simulink model "controller"  (Simulink 7.5)
settings: Solver=FixedStepDiscrete  SolverMode=SingleTasking  StartTime=0.0  StopTime=10.0  FixedStep=0.01  RelTol=1e-3
InitFcn:
  | controller_params
undefined symbols (not defined in the file): C_d_sea_surge, d_prop, DiscIntNeverNeededParam, InitialPoint, IPStar, ISA_g, K_t, mass, MaxDwnPthStar, OC2max, phi_0, rho_w, switchDistance, tanIntercept, TStar, Turn2Track, wheelbase
libraries: simulink x8, uSimLib x3, aerolibconvert2 x2, simulink_need_slupdate x1
settings Model: Creator=Bryant  LastModifiedBy=Bryant
settings DataIOCC: LimitDataPoints=off  SaveOutput=off  SignalLogging=off  DSMLogging=off  SaveTime=off
settings OptimizationCC: InlineParams=on  InlineInvariantSignals=on  InitFltsAndDblsToZero=on  EfficientFloat2IntCast=on  SimCompilerOptimization=On
settings HardwareCC: ProdBitPerInt=16  ProdIntDivRoundTo=Zero  ProdEndianess=LittleEndian  ProdWordSize=16  ProdHWDeviceType=16-bit Generic
settings ModelReferenceCC: EnableParallelModelReferenceBuilds=on  ParallelModelReferenceMATLABWorkerInit=Copy Base Workspace  ModelReferenceNumInstancesAllowed=Single
settings RTWCC: SystemTargetFile=dspic.tlc  MakeCommand=make_CreateMPLAB  TemplateMakefile=dspic_pic30_gcc.tmf  PostCodeGenCommand=dsPIC_Compile()  Description=Embedded Target for Microchip dsPIC (real-time)  ProcessScript=dspic_make_rtw_hook
settings CodeAppCC: MaxIdLength=80
settings STFCustomTargetCC: IncludeMdlTerminateFcn=off  GeneratePreprocessorConditionals=Disable all  SupportNonInlinedSFcns=off  SystemTargetFile=dspic.tlc
settings ERTTargetCC: MultiwordLength=2048  ParMdlRefBuildCompliant=off  CompOptLevelCompliant=off  IncludeMdlTerminateFcn=off  GeneratePreprocessorConditionals=Disable all  CombineOutputUpdateFcns=off  ERTFirstTimeCompliant=off  ERTCustomFileBanners=off  SupportContinuousTime=on  ModelStepFunctionPrototypeControlCompliant=off  CPPClassGenCompliant=off  ExtModeMexFile=ext_serial_win32_comm  InlinedParameterPlacement=NonHierarchical  ERTSrcFileBannerTemplate=dsPIC_code_template.cgt  ERTHdrFileBannerTemplate=dsPIC_code_template.cgt  ERTDataSrcFileTemplate=dsPIC_code_template.cgt  ERTDataHdrFileTemplate=dsPIC_code_template.cgt  ERTCustomFileTemplate=dsPIC_main.tlc  ConvertIfToSwitch=off
settings CustomProperty: DataType=string  Value=C:\PROGRA~1\MATLAB\R2010a\bin\win64\gmake

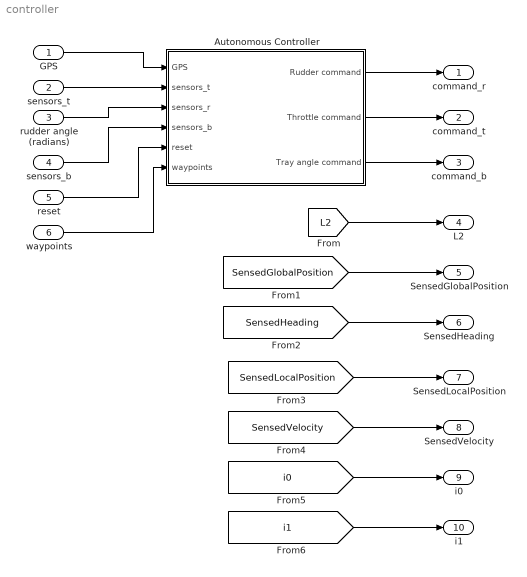
== system controller ==
  GPS : Inport  UseBusObject=on
      settings: BusObject=GpsBus
  sensors_t : Inport  Port=2  PortDimensions=1  DataType=int16  OutDataTypeStr=int16
  rudder angle (radians) : Inport  Port=3  PortDimensions=1  DataType=single  OutDataTypeStr=single
  sensors_b : Inport  Port=4  UseBusObject=on
      settings: BusObject=BallastSensorBus
  reset : Inport  Port=5  PortDimensions=1  DataType=boolean  OutDataTypeStr=boolean
  waypoints : Inport  Port=6  PortDimensions=[11,3]  DataType=int32  OutDataTypeStr=int32  Interpolate=off
  Autonomous Controller : Subsystem
  command_r : Outport  UseBusObject=on
      settings: BusObject=RudderOutBus
  command_t : Outport  Port=2  UseBusObject=on
      settings: BusObject=ThrottleOutBus
  command_b : Outport  Port=3  UseBusObject=on
      settings: BusObject=BallastOutBus
  L2 : Outport  Port=4  PortDimensions=3  DataType=single  OutDataTypeStr=single
      settings: BusObject=BallastOutBus
  SensedGlobalPosition : Outport  Port=5  PortDimensions=3  DataType=single  OutDataTypeStr=single
      settings: BusObject=BallastOutBus
  SensedHeading : Outport  Port=6  PortDimensions=1  DataType=single  OutDataTypeStr=single
      settings: BusObject=BallastOutBus
  SensedLocalPosition : Outport  Port=7  PortDimensions=3  DataType=single  OutDataTypeStr=single
      settings: BusObject=BallastOutBus
  SensedVelocity : Outport  Port=8  PortDimensions=3  DataType=single  OutDataTypeStr=single
      settings: BusObject=BallastOutBus
  i0 : Outport  Port=9  PortDimensions=1  DataType=int8  OutDataTypeStr=int8
      settings: BusObject=BallastOutBus
  i1 : Outport  Port=10  PortDimensions=1  DataType=int8  OutDataTypeStr=int8
      settings: BusObject=BallastOutBus
  wires:
  Autonomous Controller/1(Rudder command) -> command_r/1
  Autonomous Controller/2(Throttle command) -> command_t/1
  Autonomous Controller/3(Tray angle command) -> command_b/1
  GPS/1 -> Autonomous Controller/1(GPS)
  sensors_t/1 -> Autonomous Controller/2(sensors_t)
  rudder angle (radians)/1 -> Autonomous Controller/3(sensors_r)
  sensors_b/1 -> Autonomous Controller/4(sensors_b)
  reset/1 -> Autonomous Controller/5(reset)
  waypoints/1 -> Autonomous Controller/6(waypoints)
  [L2] -> L2/1
  [SensedGlobalPosition] -> SensedGlobalPosition/1
  [SensedHeading] -> SensedHeading/1
  [SensedLocalPosition] -> SensedLocalPosition/1
  [SensedVelocity] -> SensedVelocity/1
  [i0] -> i0/1
  [i1] -> i1/1

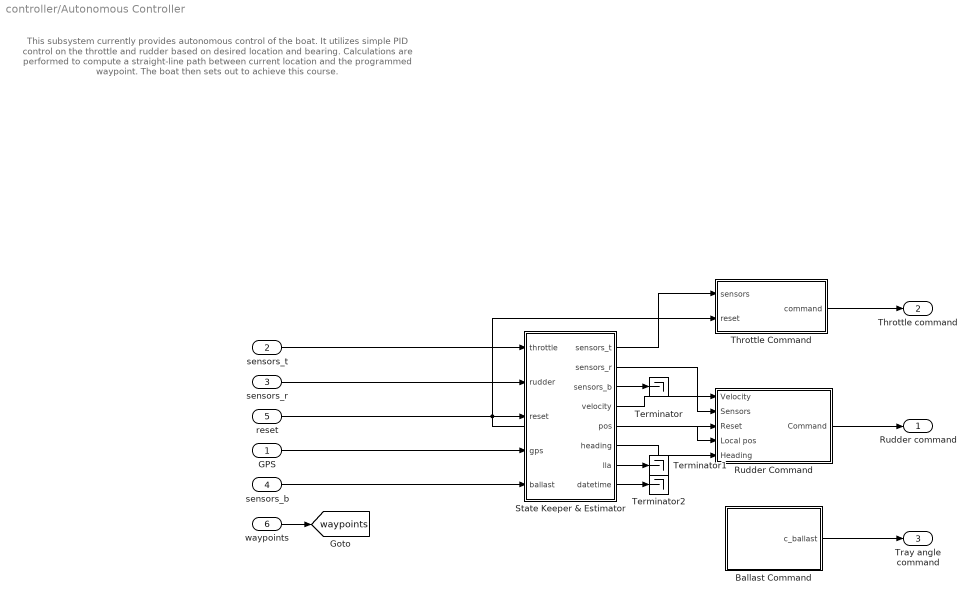
== system controller/Autonomous Controller ==
  note: This subsystem currently provides autonomous control of the boat. It utilizes simple PID control
      | on the throttle and rudder based on desired location and bearing. Calculations are performed
      | to compute a straight-line path between current location and the programmed waypoint. The
      | boat then sets out to achieve this course.
  GPS : Inport  OutDataType=sfix(16)  OutScaling=2^0
  sensors_t : Inport  Port=2  OutDataType=sfix(16)  OutScaling=2^0
  sensors_r : Inport  Port=3  OutDataType=sfix(16)  OutScaling=2^0
  sensors_b : Inport  Port=4  OutDataType=sfix(16)  OutScaling=2^0
  reset : Inport  Port=5  OutDataType=sfix(16)  OutScaling=2^0
  waypoints : Inport  Port=6  OutDataType=sfix(16)  OutScaling=2^0
  Ballast Command : Subsystem
  Rudder Command : Subsystem
  State Keeper & Estimator : Subsystem
  Terminator : Terminator
  Terminator1 : Terminator
  Terminator2 : Terminator
  Throttle Command : Subsystem
  Rudder command : Outport  OutDataType=sfix(16)  OutScaling=2^0
  Throttle command : Outport  Port=2  OutDataType=sfix(16)  OutScaling=2^0
  Tray angle command : Outport  Port=3  OutDataType=sfix(16)  OutScaling=2^0
  tag scope: waypoints=global
  wires:
  sensors_t/1 -> State Keeper & Estimator/1(throttle)
  sensors_r/1 -> State Keeper & Estimator/2(rudder)
  sensors_b/1 -> State Keeper & Estimator/5(ballast)
  Ballast Command/1(c_ballast) -> Tray angle command/1
  Rudder Command/1(Command) -> Rudder command/1
  Throttle Command/1(command) -> Throttle command/1
  GPS/1 -> State Keeper & Estimator/4(gps)
  State Keeper & Estimator/4(velocity) -> Rudder Command/1(Velocity)
  State Keeper & Estimator/2(sensors_r) -> Rudder Command/2(Sensors)
  State Keeper & Estimator/1(sensors_t) -> Throttle Command/1(sensors)
  State Keeper & Estimator/5(pos) -> Rudder Command/4(Local pos)
  reset/1 -> State Keeper & Estimator/3(reset), Throttle Command/2(reset), Rudder Command/3(Reset)
  waypoints/1 -> [waypoints]
  State Keeper & Estimator/6(heading) -> Rudder Command/5(Heading)
  State Keeper & Estimator/3(sensors_b) -> Terminator/1
  State Keeper & Estimator/7(lla) -> Terminator1/1
  State Keeper & Estimator/8(datetime) -> Terminator2/1

== system controller/Autonomous Controller/Ballast Command ==
  Bus Creator : BusCreator  Inputs=2
  Constant : Constant  Value=0  OutDataTypeMode=boolean  OutDataType=fixdt(1, 16)  OutScaling=2^0  OutDataTypeStr=boolean
  Constant1 : Constant  Value=0  OutDataTypeMode=boolean  OutDataType=fixdt(1, 16)  OutScaling=2^0  OutDataTypeStr=boolean
  c_ballast : Outport
  wires:
  Bus Creator/1 -> c_ballast/1
  Constant/1 -> Bus Creator/1  "enable"
  Constant1/1 -> Bus Creator/2  "direction"

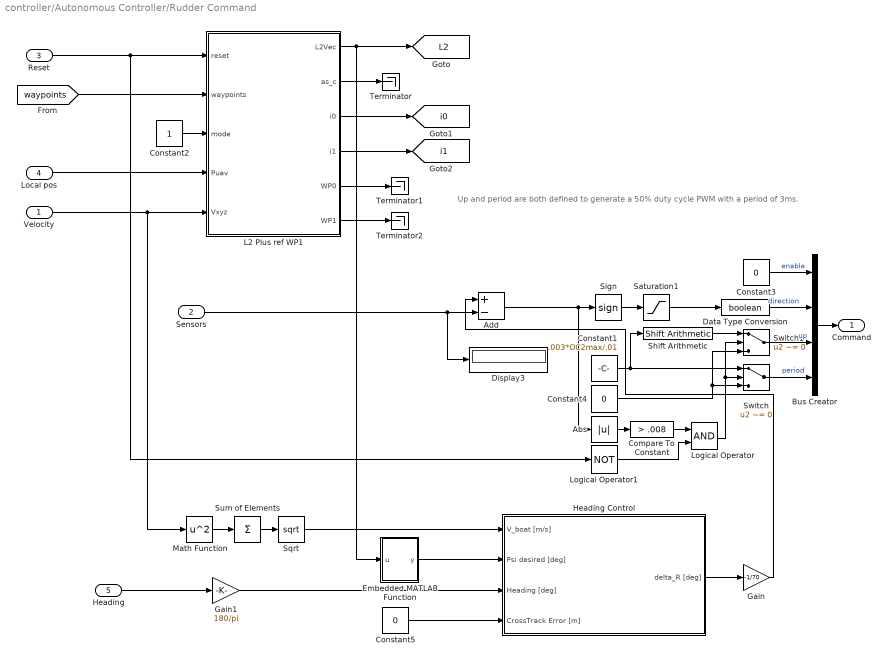
== system controller/Autonomous Controller/Rudder Command ==
  note: Up and period are both defined to generate a 50% duty cycle PWM with
      | a period of 3ms.
  Velocity : Inport
  Sensors : Inport  Port=2
  Reset : Inport  Port=3
  Local pos : Inport  Port=4
  Heading : Inport  Port=5
  Abs : Abs  OutDataType=fixdt(1, 16)  OutScaling=2^0
  Add : Sum  Inputs=+-  OutDataType=fixdt(1, 16)  OutScaling=2^-10
  Bus Creator : BusCreator
  Compare To Constant : simulink/Logic and Bit Operations/Compare To Constant  SystemSampleTime=-1  relop=>  const=.008  LogicOutDataTypeMode=boolean
  Constant1 : Constant  Value=.003*OC2max/.01  OutDataTypeMode=uint16  OutDataType=sfix(16)  OutScaling=2^0  OutDataTypeStr=uint16
  Constant2 : Constant  OutDataTypeMode=uint8  OutDataType=sfix(16)  OutScaling=2^0  OutDataTypeStr=uint8
  Constant3 : Constant  Value=0  OutDataTypeMode=boolean  OutDataType=sfix(16)  OutScaling=2^0  OutDataTypeStr=boolean
  Constant4 : Constant  Value=0  OutDataTypeMode=uint16  OutDataType=sfix(16)  OutScaling=2^0  OutDataTypeStr=uint16
  Constant5 : Constant  Value=0  OutDataTypeMode=uint8  OutDataType=sfix(16)  OutScaling=2^0  OutDataTypeStr=uint8
  Data Type Conversion : DataTypeConversion  OutDataTypeMode=boolean  OutDataType=fixdt(1, 16)  OutScaling=2^0  OutDataTypeStr=boolean  RndMeth=Simplest
  Display3 : Display
  Embedded MATLAB Function : Stateflow chart  TreatAsAtomicUnit=on
  Gain : Gain  Gain=-1/70  ParameterDataType=fixdt(1, 16)  ParameterScaling=2^0  OutDataType=fixdt(1, 16)  OutScaling=2^0
  Gain1 : Gain  Gain=180/pi  ParameterDataType=fixdt(1, 16)  ParameterScaling=2^0  OutDataType=fixdt(1, 16)  OutScaling=2^0
  Heading Control : Subsystem
  L2 Plus ref WP1 : Stateflow chart  TreatAsAtomicUnit=on
  Logical Operator : Logic  AllPortsSameDT=off  OutDataTypeMode=boolean  LogicDataType=fixdt(0, 8)  OutDataTypeStr=boolean
  Logical Operator1 : Logic  Operator=NOT  Inputs=1  AllPortsSameDT=off  OutDataTypeMode=boolean  LogicDataType=fixdt(0, 8)  OutDataTypeStr=boolean
  Math Function : Math  Operator=square  OutDataType=fixdt(1, 16)  OutScaling=2^0  SaturateOnIntegerOverflow=on
  Saturation1 : Saturate  UpperLimit=1  LowerLimit=0  OutDataTypeStr=Inherit: Inherit via back propagation
  Shift Arithmetic : simulink/Logic and Bit Operations/Shift Arithmetic  SystemSampleTime=-1  nBitShiftRight=1  nBinPtShiftRight=0
  Sign : Signum
  Sqrt : Sqrt  SaturateOnIntegerOverflow=on
  Sum of Elements : Sum  Inputs=+  OutDataType=fixdt(1, 16)  OutScaling=2^-10
  Switch : Switch  Criteria=u2 ~= 0  OutDataType=fixdt(1, 16)  OutScaling=2^0
  Switch1 : Switch  Criteria=u2 ~= 0  OutDataType=fixdt(1, 16)  OutScaling=2^0
  Terminator : Terminator
  Terminator1 : Terminator
  Terminator2 : Terminator
  Command : Outport
  tag scope: L2=global, i0=global, i1=global
  wires:
  Data Type Conversion/1 -> Bus Creator/2  "direction"
  Sensors/1 -> Display3/1, Add/2
  Bus Creator/1 -> Command/1
  Saturation1/1 -> Data Type Conversion/1
  Sign/1 -> Saturation1/1
  Constant2/1 -> L2 Plus ref WP1/3(mode)
  L2 Plus ref WP1/1(L2Vec) -> [L2], Embedded MATLAB Function/1(u)
  Velocity/1 -> L2 Plus ref WP1/5(Vxyz), Math Function/1
  Constant3/1 -> Bus Creator/1  "enable"
  Constant1/1 -> Shift Arithmetic/1, Switch/1
  Abs/1 -> Compare To Constant/1
  Shift Arithmetic/1 -> Switch1/1
  Switch/1 -> Bus Creator/4  "period"
  Switch1/1 -> Bus Creator/3  "up"
  Constant4/1 -> Switch/3, Switch1/3
  Reset/1 -> L2 Plus ref WP1/1(reset), Logical Operator1/1
  Local pos/1 -> L2 Plus ref WP1/4(Puav)
  L2 Plus ref WP1/3(i0) -> [i0]
  L2 Plus ref WP1/4(i1) -> [i1]
  Compare To Constant/1 -> Logical Operator/1
  Logical Operator/1 -> Switch/2, Switch1/2
  Logical Operator1/1 -> Logical Operator/2
  [waypoints] -> L2 Plus ref WP1/2(waypoints)
  Heading/1 -> Gain1/1
  Constant5/1 -> Heading Control/4(CrossTrack Error [m])
  Sqrt/1 -> Heading Control/1(V_boat [m/s])
  Math Function/1 -> Sum of Elements/1
  Sum of Elements/1 -> Sqrt/1
  Heading Control/1(delta_R [deg]) -> Gain/1
  Gain/1 -> Add/1
  Gain1/1 -> Heading Control/3(Heading [deg])
  Embedded MATLAB Function/1(y) -> Heading Control/2(Psi desired [deg])
  Add/1 -> Sign/1, Abs/1
  L2 Plus ref WP1/2(as_c) -> Terminator/1
  L2 Plus ref WP1/5(WP0) -> Terminator1/1
  L2 Plus ref WP1/6(WP1) -> Terminator2/1

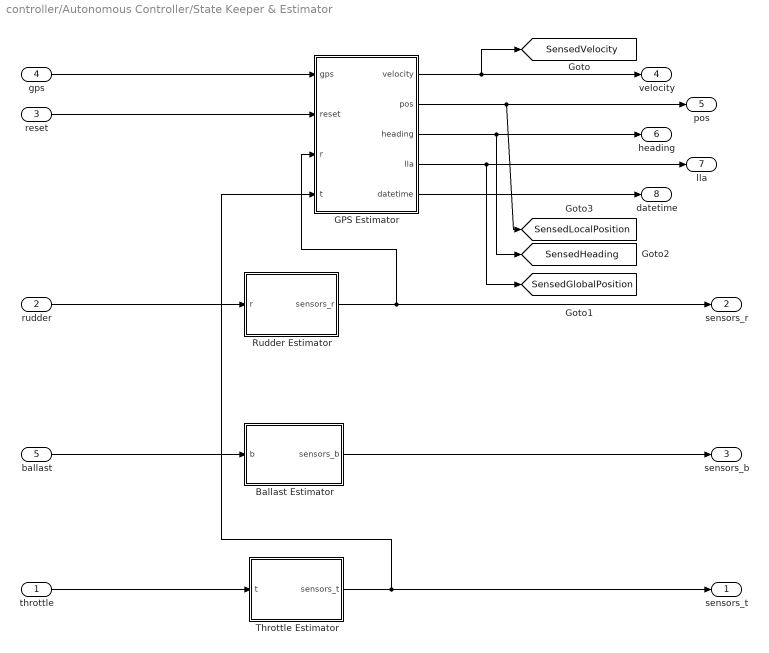
== system controller/Autonomous Controller/State Keeper & Estimator ==
  throttle : Inport
  rudder : Inport  Port=2
  reset : Inport  Port=3
  gps : Inport  Port=4
  ballast : Inport  Port=5
  Ballast Estimator : Subsystem
  GPS Estimator : Subsystem
  Rudder Estimator : Subsystem
  Throttle Estimator : Subsystem
  sensors_t : Outport
  sensors_r : Outport  Port=2
  sensors_b : Outport  Port=3
  velocity : Outport  Port=4
  pos : Outport  Port=5
  heading : Outport  Port=6
  lla : Outport  Port=7
  datetime : Outport  Port=8
  tag scope: SensedGlobalPosition=global, SensedHeading=global, SensedLocalPosition=global, SensedVelocity=global
  wires:
  rudder/1 -> Rudder Estimator/1(r)
  ballast/1 -> Ballast Estimator/1(b)
  throttle/1 -> Throttle Estimator/1(t)
  reset/1 -> GPS Estimator/2(reset)
  GPS Estimator/1(velocity) -> velocity/1, [SensedVelocity]
  gps/1 -> GPS Estimator/1(gps)
  GPS Estimator/2(pos) -> pos/1, [SensedLocalPosition]
  GPS Estimator/3(heading) -> heading/1, [SensedHeading]
  GPS Estimator/4(lla) -> [SensedGlobalPosition], lla/1
  GPS Estimator/5(datetime) -> datetime/1
  Rudder Estimator/1(sensors_r) -> sensors_r/1, GPS Estimator/3(r)
  Ballast Estimator/1(sensors_b) -> sensors_b/1
  Throttle Estimator/1(sensors_t) -> sensors_t/1, GPS Estimator/4(t)

== system controller/Autonomous Controller/Throttle Command ==
  sensors : Inport
  reset : Inport  Port=2
  Bus Creator : BusCreator
  Constant1 : Constant  Value=0  OutDataTypeMode=int16  OutDataType=sfix(16)  OutScaling=2^0  OutDataTypeStr=int16
  Constant5 : Constant  Value=1000  OutDataTypeMode=int16  OutDataType=sfix(16)  OutScaling=2^0  OutDataTypeStr=int16
  Mux Everything : Subsystem
  Switch : Switch  Criteria=u2 > Threshold  OutDataType=fixdt(1, 16)  OutScaling=2^0
  Terminator : Terminator
  Trigger Events : Subsystem
  command : Outport  OutDataType=sfix(16)  OutScaling=2^0
  wires:
  sensors/1 -> Terminator/1
  Bus Creator/1 -> command/1
  Trigger Events/1(Change Speed) -> Mux Everything/1(speed)
  Trigger Events/3(Enable) -> Mux Everything/3(enable)
  Trigger Events/2(Disable) -> Mux Everything/2(disable)
  reset/1 -> Trigger Events/2(Reset), Switch/2
  Mux Everything/1(iden) -> Bus Creator/1  "identifier"
  Mux Everything/2(data) -> Bus Creator/2  "data"
  Mux Everything/3(size) -> Bus Creator/3  "size"
  Mux Everything/4(trig) -> Bus Creator/4  "trigger"
  Switch/1 -> Mux Everything/4(Throttle), Trigger Events/1(RC Throttle)
  Constant1/1 -> Switch/1
  Constant5/1 -> Switch/3

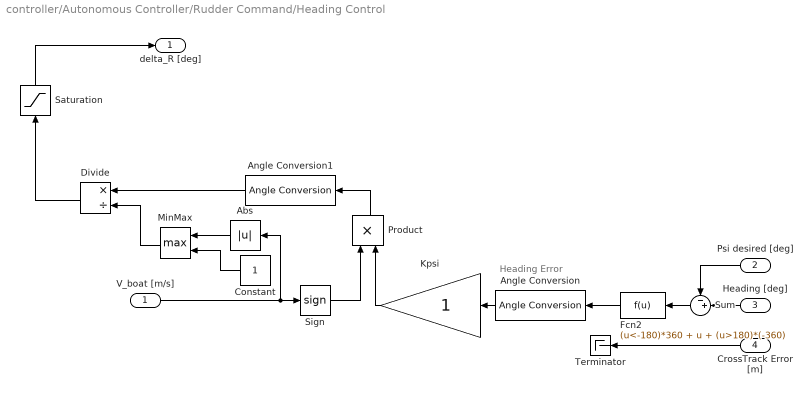
== system controller/Autonomous Controller/Rudder Command/Heading Control ==
  note: Heading Error
  V_boat [m/s] : Inport  OutDataType=sfix(16)  OutScaling=2^0
  Psi desired [deg] : Inport  Port=2  OutDataType=sfix(16)  OutScaling=2^0
  Heading [deg] : Inport  Port=3  OutDataType=sfix(16)  OutScaling=2^0
  CrossTrack Error [m] : Inport  Port=4  OutDataType=sfix(16)  OutScaling=2^0
  Abs : Abs
  Angle Conversion : aerolibconvert2/Angle Conversion  SystemSampleTime=-1  IU=deg  OU=rad
  Angle Conversion1 : aerolibconvert2/Angle Conversion  SystemSampleTime=-1  IU=rad  OU=deg
  Constant : Constant  OutDataType=sfix(16)  OutScaling=2^0
  Divide : Product  Inputs=*/  OutDataType=sfix(16)  OutScaling=2^-10
  Fcn2 : Fcn  Expr=(u<-180)*360 + u + (u>180)*(-360)
  Kpsi : Gain  ParameterDataType=sfix(16)  ParameterScaling=2^0  OutDataType=sfix(16)  OutScaling=2^0
  MinMax : MinMax  Function=max  Inputs=2  OutDataType=sfix(16)  OutScaling=2^0
  Product : Product  OutDataType=sfix(16)  OutScaling=2^0  RndMeth=Zero
  Saturation : Saturate  UpperLimit=70  LowerLimit=-70
  Sign : Signum
  Sum : Sum  Inputs=-+|  OutDataType=sfix(16)  OutScaling=2^0
  Terminator : Terminator
  delta_R [deg] : Outport  OutDataType=sfix(16)  OutScaling=2^0
  wires:
  Sum/1 -> Fcn2/1
  Heading [deg]/1 -> Sum/2
  Psi desired [deg]/1 -> Sum/1
  CrossTrack Error [m]/1 -> Terminator/1
  MinMax/1 -> Divide/2
  Saturation/1 -> delta_R [deg]/1
  Constant/1 -> MinMax/2
  Abs/1 -> MinMax/1
  Divide/1 -> Saturation/1
  Angle Conversion1/1 -> Divide/1
  Sign/1 -> Product/1
  Kpsi/1 -> Product/2
  Product/1 -> Angle Conversion1/1
  V_boat [m/s]/1 -> Sign/1, Abs/1
  Angle Conversion/1 -> Kpsi/1
  Fcn2/1 -> Angle Conversion/1

== system controller/Autonomous Controller/State Keeper & Estimator/Ballast Estimator ==
  b : Inport
  Bus Selector1 : BusSelector  OutputSignals=position
  sensors_b : Outport
  wires:
  b/1 -> Bus Selector1/1
  Bus Selector1/1 -> sensors_b/1  "<position>"

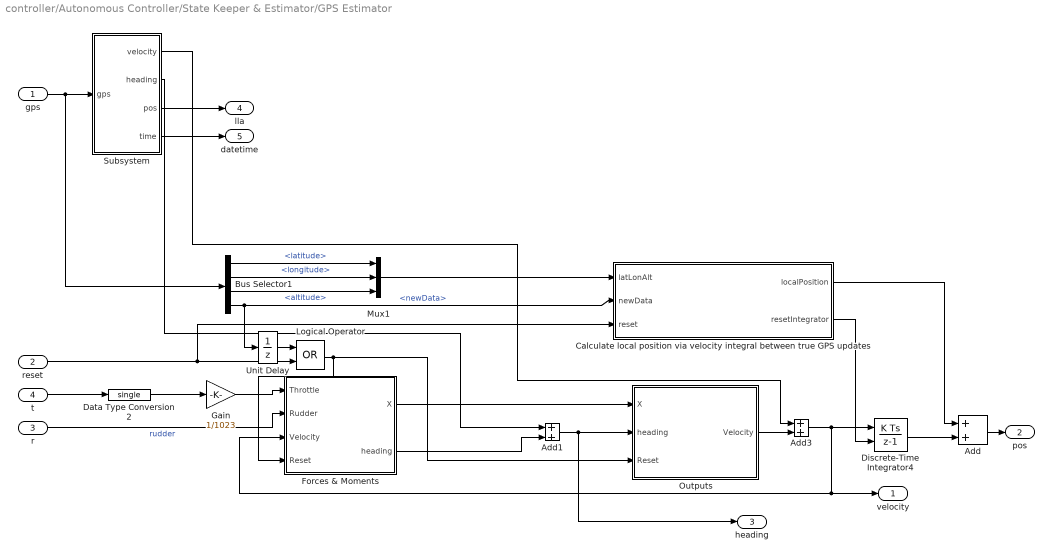
== system controller/Autonomous Controller/State Keeper & Estimator/GPS Estimator ==
  gps : Inport
  reset : Inport  Port=2  OutDataType=fixdt(1, 16)  OutScaling=2^0
  r : Inport  Port=3  OutDataType=fixdt(1, 16)  OutScaling=2^0
  t : Inport  Port=4  OutDataType=fixdt(1, 16)  OutScaling=2^0
  Add : Sum  OutDataType=fixdt(1, 16)  OutScaling=2^-10
  Add1 : Sum  OutDataType=fixdt(1, 16)  OutScaling=2^-10
  Add3 : Sum  OutDataType=fixdt(1, 16)  OutScaling=2^-10
  Bus Selector1 : BusSelector  OutputSignals=latitude,longitude,altitude,newData
  Calculate local position via velocity integral between true GPS updates : Stateflow chart  TreatAsAtomicUnit=on
  Data Type Conversion2 : DataTypeConversion  OutDataTypeMode=single  OutDataType=sfix(16)  OutScaling=2^0  OutDataTypeStr=single  LockScale=on
  Discrete-Time Integrator4 : DiscreteIntegrator  ExternalReset=level  SampleTime=-1  OutDataType=fixdt(1, 16)  OutScaling=2^0  ICPrevOutput=DiscIntNeverNeededParam  ICPrevScaledInput=DiscIntNeverNeededParam
  Forces & Moments : Subsystem
  Gain : Gain  Gain=1/1023  ParameterDataType=fixdt(1, 16)  ParameterScaling=2^0  OutDataType=fixdt(1, 16)  OutScaling=2^0
  Logical Operator : Logic  Operator=OR  AllPortsSameDT=off  OutDataTypeMode=boolean  LogicDataType=fixdt(0, 8)  OutDataTypeStr=boolean
  Mux1 : Mux  Inputs=3
  Outputs : Subsystem
  Subsystem : Subsystem
  Unit Delay : UnitDelay  SampleTime=-1
  velocity : Outport
  pos : Outport  Port=2
  heading : Outport  Port=3
  lla : Outport  Port=4
  datetime : Outport  Port=5
  wires:
  gps/1 -> Subsystem/1(gps), Bus Selector1/1
  Subsystem/1(velocity) -> Add3/1
  Subsystem/2(heading) -> Add1/1
  Subsystem/3(pos) -> lla/1
  Subsystem/4(time) -> datetime/1
  Forces & Moments/1(X) -> Outputs/1(X)
  r/1 -> Forces & Moments/2(Rudder)  "rudder"
  reset/1 -> Logical Operator/2, Calculate local position via velocity integral between true GPS updates/3(reset)
  Add1/1 -> Outputs/2(heading), heading/1
  Forces & Moments/2(heading) -> Add1/2
  Data Type Conversion2/1 -> Gain/1
  Gain/1 -> Forces & Moments/1(Throttle)
  t/1 -> Data Type Conversion2/1
  Discrete-Time Integrator4/1 -> Add/2
  Add/1 -> pos/1
  Bus Selector1/1 -> Mux1/1  "<latitude>"
  Bus Selector1/2 -> Mux1/2  "<longitude>"
  Bus Selector1/3 -> Mux1/3  "<altitude>"
  Bus Selector1/4 -> Calculate local position via velocity integral between true GPS updates/2(newData), Unit Delay/1  "<newData>"
  Mux1/1 -> Calculate local position via velocity integral between true GPS updates/1(latLonAlt)
  Calculate local position via velocity integral between true GPS updates/2(resetIntegrator) -> Discrete-Time Integrator4/2
  Calculate local position via velocity integral between true GPS updates/1(localPosition) -> Add/1
  Logical Operator/1 -> Outputs/3(Reset), Forces & Moments/4(Reset)
  Outputs/1(Velocity) -> Add3/2
  Add3/1 -> Discrete-Time Integrator4/1, velocity/1, Forces & Moments/3(Velocity)
  Unit Delay/1 -> Logical Operator/1

== system controller/Autonomous Controller/State Keeper & Estimator/Rudder Estimator ==
  r : Inport
  sensors_r : Outport
  wires:
  r/1 -> sensors_r/1

== system controller/Autonomous Controller/State Keeper & Estimator/Throttle Estimator ==
  t : Inport
  sensors_t : Outport
  wires:
  t/1 -> sensors_t/1

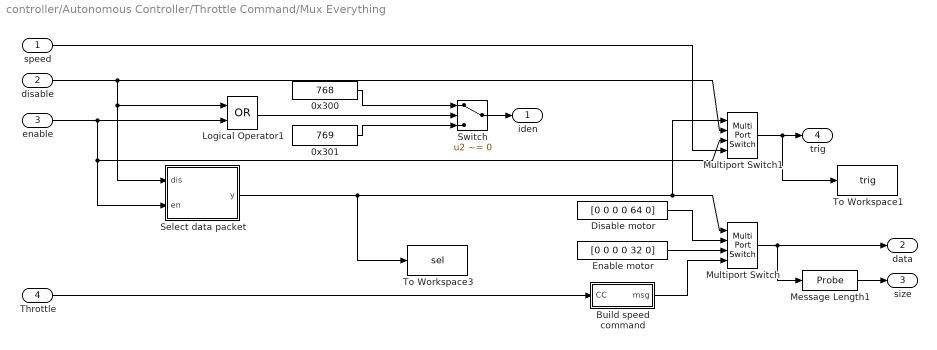
== system controller/Autonomous Controller/Throttle Command/Mux Everything ==
  speed : Inport  OutDataType=sfix(16)  OutScaling=2^0
  disable : Inport  Port=2  OutDataType=sfix(16)  OutScaling=2^0
  enable : Inport  Port=3  OutDataType=sfix(16)  OutScaling=2^0
  Throttle : Inport  Port=4  OutDataType=sfix(16)  OutScaling=2^0
  0x300 : Constant  Value=768  OutDataTypeMode=uint32  OutDataType=sfix(16)  OutScaling=2^0  OutDataTypeStr=uint32
  0x301 : Constant  Value=769  OutDataTypeMode=uint32  OutDataType=sfix(16)  OutScaling=2^0  OutDataTypeStr=uint32
  Build speed command : Subsystem
  Disable motor : Constant  Value=[0 0 0 0 64 0]  OutDataTypeMode=uint8  OutDataType=sfix(16)  OutScaling=2^0  OutDataTypeStr=uint8
  Enable motor : Constant  Value=[0 0 0 0 32 0]  OutDataTypeMode=uint8  OutDataType=sfix(16)  OutScaling=2^0  OutDataTypeStr=uint8
  Logical Operator1 : Logic  Operator=OR  AllPortsSameDT=off  OutDataTypeMode=boolean  OutDataTypeStr=boolean
  Message Length1 : Probe  ProbeSampleTime=off  ProbeComplexSignal=off  ProbeWidthDataType=uint8
  Multiport Switch : MultiPortSwitch  zeroidx=off
  Multiport Switch1 : MultiPortSwitch  zeroidx=off
  Select data packet : Stateflow chart  TreatAsAtomicUnit=on
  Switch : Switch  Criteria=u2 ~= 0
  To Workspace1 : ToWorkspace  VariableName=trig  SampleTime=-1  SaveFormat=Array
  To Workspace3 : ToWorkspace  VariableName=sel  SampleTime=-1  SaveFormat=Array
  iden : Outport  OutDataType=sfix(16)  OutScaling=2^0
  data : Outport  Port=2  OutDataType=sfix(16)  OutScaling=2^0
  size : Outport  Port=3  OutDataType=sfix(16)  OutScaling=2^0
  trig : Outport  Port=4  OutDataType=sfix(16)  OutScaling=2^0
  wires:
  Enable motor/1 -> Multiport Switch/3
  Disable motor/1 -> Multiport Switch/2
  Throttle/1 -> Build speed command/1(CC)
  Multiport Switch/1 -> Message Length1/1, data/1
  Message Length1/1 -> size/1
  0x300/1 -> Switch/1
  0x301/1 -> Switch/3
  Switch/1 -> iden/1
  disable/1 -> Logical Operator1/1, Select data packet/1(dis), Multiport Switch1/2
  enable/1 -> Logical Operator1/2, Select data packet/2(en), Multiport Switch1/3
  Logical Operator1/1 -> Switch/2
  Select data packet/1(y) -> Multiport Switch/1, Multiport Switch1/1, To Workspace3/1
  Multiport Switch1/1 -> trig/1, To Workspace1/1
  speed/1 -> Multiport Switch1/4
  Build speed command/1(msg) -> Multiport Switch/4

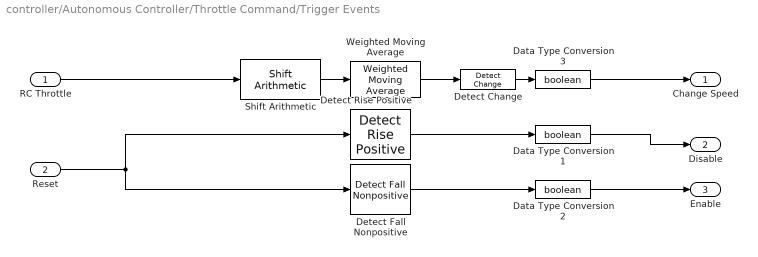
== system controller/Autonomous Controller/Throttle Command/Trigger Events ==
  RC Throttle : Inport  OutDataType=sfix(16)  OutScaling=2^0
  Reset : Inport  Port=2  OutDataType=sfix(16)  OutScaling=2^0
  Data Type Conversion1 : DataTypeConversion  OutDataTypeMode=boolean  OutDataType=sfix(16)  OutScaling=2^0  OutDataTypeStr=boolean
  Data Type Conversion2 : DataTypeConversion  OutDataTypeMode=boolean  OutDataType=sfix(16)  OutScaling=2^0  OutDataTypeStr=boolean
  Data Type Conversion3 : DataTypeConversion  OutDataTypeMode=boolean  OutDataType=sfix(16)  OutScaling=2^0  OutDataTypeStr=boolean
  Detect Change : simulink/Logic and Bit Operations/Detect Change  SystemSampleTime=-1  vinit=0
  Detect Fall Nonpositive : simulink/Logic and Bit Operations/Detect Fall Nonpositive  SystemSampleTime=-1  vinit=0
  Detect Rise Positive : simulink/Logic and Bit Operations/Detect Rise Positive  SystemSampleTime=-1  vinit=0
  Shift Arithmetic : simulink/Logic and Bit Operations/Shift Arithmetic  SystemSampleTime=-1  nBitShiftRight=2  nBinPtShiftRight=0
  Weighted Moving Average : simulink_need_slupdate/Weighted Moving Average  mgainval=[.5 .5]  vinit=0.0  samptime=-1  OutDataTypeStr=Inherit: Inherit via back propagation  OutDataType=sfix(16)  OutScaling=2^-10  DoSatur=off  GainDataType=uint(16)  MatRadixGroup=Best Precision: Matrix-wise  GainScaling=2^-10
  Change Speed : Outport  OutDataType=sfix(16)  OutScaling=2^0
  Disable : Outport  Port=2  OutDataType=sfix(16)  OutScaling=2^0
  Enable : Outport  Port=3  OutDataType=sfix(16)  OutScaling=2^0
  wires:
  RC Throttle/1 -> Shift Arithmetic/1
  Detect Change/1 -> Data Type Conversion3/1
  Weighted Moving Average/1 -> Detect Change/1
  Shift Arithmetic/1 -> Weighted Moving Average/1
  Reset/1 -> Detect Fall Nonpositive/1, Detect Rise Positive/1
  Detect Fall Nonpositive/1 -> Data Type Conversion2/1
  Detect Rise Positive/1 -> Data Type Conversion1/1
  Data Type Conversion3/1 -> Change Speed/1
  Data Type Conversion2/1 -> Enable/1
  Data Type Conversion1/1 -> Disable/1

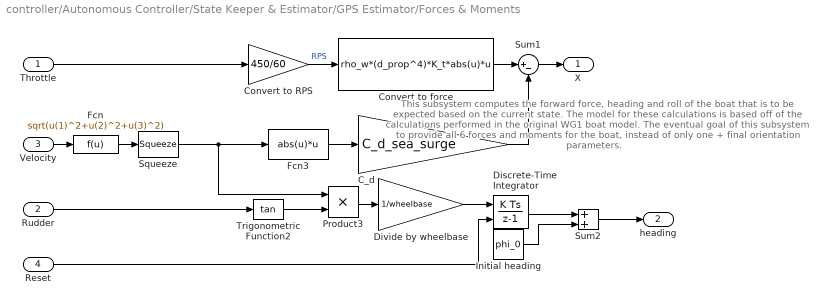
== system controller/Autonomous Controller/State Keeper & Estimator/GPS Estimator/Forces & Moments ==
  note: This subsystem computes the forward force, heading and roll of the boat that
      | is to be expected based on the current state. The model for these calculations
      | is based off of the calculations performed in the original WG1 boat model.
      |
      | The eventual goal of this subsystem to provide all 6 forces and moments for the
      | boat, instead of only one + final orientation parameters.
  Throttle : Inport  OutDataType=sfix(16)  OutScaling=2^0
  Rudder : Inport  Port=2  OutDataType=sfix(16)  OutScaling=2^0
  Velocity : Inport  Port=3  OutDataType=sfix(16)  OutScaling=2^0
  Reset : Inport  Port=4  OutDataType=sfix(16)  OutScaling=2^0
  C_d : Gain  Gain=C_d_sea_surge  ParameterDataType=sfix(16)  ParameterScaling=2^0  OutDataType=sfix(16)  OutScaling=2^0
  Convert to RPS : Gain  Gain=450/60  ParameterDataType=sfix(16)  ParameterScaling=2^0  OutDataType=sfix(16)  OutScaling=2^0
  Convert to force : Fcn  Expr=rho_w*(d_prop^4)*K_t*abs(u)*u
  Discrete-Time Integrator : DiscreteIntegrator  ExternalReset=level  SampleTime=-1  OutDataType=fixdt(1, 16)  OutScaling=2^0  ICPrevOutput=DiscIntNeverNeededParam  ICPrevScaledInput=DiscIntNeverNeededParam
  Divide by wheelbase : Gain  Gain=1/wheelbase  ParameterDataType=sfix(16)  ParameterScaling=2^0  OutDataType=sfix(16)  OutScaling=2^0
  Fcn : Fcn  Expr=sqrt(u(1)^2+u(2)^2+u(3)^2)
  Fcn3 : Fcn  Expr=abs(u)*u
  Initial heading : Constant  Value=phi_0  OutDataTypeMode=single  OutDataType=sfix(16)  OutScaling=2^0  OutDataTypeStr=single
  Product3 : Product  OutDataType=sfix(16)  OutScaling=2^0  RndMeth=Zero
  Squeeze : Squeeze
  Sum1 : Sum  Inputs=|+-  OutDataType=sfix(16)  OutScaling=2^0
  Sum2 : Sum  OutDataType=sfix(16)  OutScaling=2^0
  Trigonometric Function2 : Trigonometry  Operator=tan  OutputSignalType=real
  X : Outport  OutDataType=sfix(16)  OutScaling=2^0
  heading : Outport  Port=2  OutDataType=sfix(16)  OutScaling=2^0
  wires:
  Sum2/1 -> heading/1
  Initial heading/1 -> Sum2/2
  Discrete-Time Integrator/1 -> Sum2/1
  Divide by wheelbase/1 -> Discrete-Time Integrator/1
  Product3/1 -> Divide by wheelbase/1
  Trigonometric Function2/1 -> Product3/2
  Rudder/1 -> Trigonometric Function2/1
  Fcn/1 -> Squeeze/1
  Sum1/1 -> X/1
  Throttle/1 -> Convert to RPS/1
  Velocity/1 -> Fcn/1
  Convert to force/1 -> Sum1/1
  C_d/1 -> Sum1/2
  Fcn3/1 -> C_d/1
  Convert to RPS/1 -> Convert to force/1  "RPS"
  Reset/1 -> Discrete-Time Integrator/2
  Squeeze/1 -> Product3/1, Fcn3/1

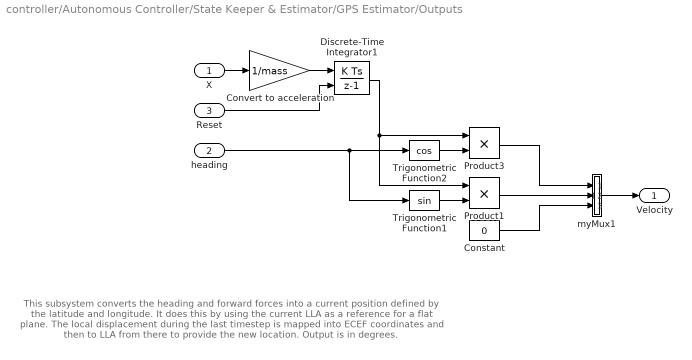
== system controller/Autonomous Controller/State Keeper & Estimator/GPS Estimator/Outputs ==
  note: This subsystem converts the heading and forward forces into a current position
      |  defined by the latitude and longitude. It does this by using the current LLA
      | as a reference for a flat plane. The local displacement during the last timestep
      | is mapped into ECEF coordinates and then to LLA from there to provide the new
      | location. Output is in degrees.
  X : Inport  OutDataType=sfix(16)  OutScaling=2^0
  heading : Inport  Port=2  OutDataType=sfix(16)  OutScaling=2^0
  Reset : Inport  Port=3  OutDataType=sfix(16)  OutScaling=2^0
  Constant : Constant  Value=0  OutDataTypeMode=single  OutDataType=fixdt(1, 16)  OutScaling=2^0  OutDataTypeStr=single
  Convert to acceleration : Gain  Gain=1/mass  ParameterDataType=sfix(16)  ParameterScaling=2^0  OutDataType=sfix(16)  OutScaling=2^0
  Discrete-Time Integrator1 : DiscreteIntegrator  ExternalReset=level  SampleTime=-1  OutDataType=fixdt(1, 16)  OutScaling=2^0  ICPrevOutput=DiscIntNeverNeededParam  ICPrevScaledInput=DiscIntNeverNeededParam
  Product1 : Product  OutDataType=sfix(16)  OutScaling=2^0  RndMeth=Zero
  Product3 : Product  OutDataType=sfix(16)  OutScaling=2^0  RndMeth=Zero
  Trigonometric Function1 : Trigonometry  OutputSignalType=real
  Trigonometric Function2 : Trigonometry  Operator=cos  OutputSignalType=real
  myMux1 : Stateflow chart  TreatAsAtomicUnit=on
  Velocity : Outport  OutDataType=sfix(16)  OutScaling=2^0
  wires:
  X/1 -> Convert to acceleration/1
  Constant/1 -> myMux1/3(u3)
  Trigonometric Function1/1 -> Product1/2
  Product1/1 -> myMux1/2(u2)
  Product3/1 -> myMux1/1(u1)
  myMux1/1(y) -> Velocity/1
  Trigonometric Function2/1 -> Product3/2
  heading/1 -> Trigonometric Function1/1, Trigonometric Function2/1
  Discrete-Time Integrator1/1 -> Product1/1, Product3/1
  Convert to acceleration/1 -> Discrete-Time Integrator1/1
  Reset/1 -> Discrete-Time Integrator1/2

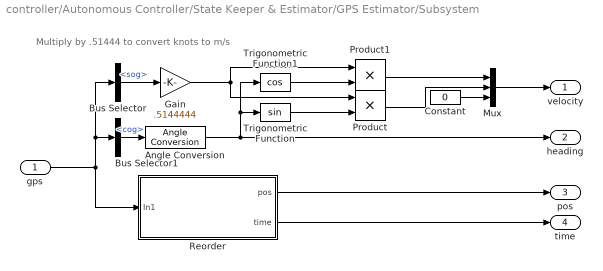
== system controller/Autonomous Controller/State Keeper & Estimator/GPS Estimator/Subsystem ==
  note: Multiply by .51444 to
      | convert knots to m/s
  gps : Inport
  Angle Conversion : uSimLib/Conversions/Angle Conversion  SystemSampleTime=-1  iu=deg  ou=rad
  Bus Selector : BusSelector  OutputSignals=sog
  Bus Selector1 : BusSelector  OutputSignals=cog
  Constant : Constant  Value=0  OutDataTypeMode=single  OutDataType=fixdt(1, 16)  OutScaling=2^0  OutDataTypeStr=single
  Gain : Gain  Gain=.5144444  ParameterDataType=fixdt(1, 16)  ParameterScaling=2^0  OutDataType=fixdt(1, 16)  OutScaling=2^0
  Mux : Mux  Inputs=3
  Product : Product  OutDataTypeMode=single  OutDataType=fixdt(1, 16)  OutScaling=2^0  OutDataTypeStr=single  RndMeth=Zero
  Product1 : Product  OutDataTypeMode=single  OutDataType=fixdt(1, 16)  OutScaling=2^0  OutDataTypeStr=single  RndMeth=Zero
  Reorder : Subsystem
  Trigonometric Function : Trigonometry
  Trigonometric Function1 : Trigonometry  Operator=cos
  velocity : Outport
  heading : Outport  Port=2
  pos : Outport  Port=3
  time : Outport  Port=4
  wires:
  Reorder/2(time) -> time/1
  Reorder/1(pos) -> pos/1
  Bus Selector/1 -> Gain/1  "<sog>"
  Angle Conversion/1 -> Trigonometric Function1/1, Trigonometric Function/1, heading/1
  Mux/1 -> velocity/1
  Constant/1 -> Mux/3
  Product/1 -> Mux/2
  Product1/1 -> Mux/1
  Trigonometric Function1/1 -> Product1/2
  Trigonometric Function/1 -> Product/2
  Bus Selector1/1 -> Angle Conversion/1  "<cog>"
  gps/1 -> Bus Selector1/1, Bus Selector/1, Reorder/1(In1)
  Gain/1 -> Product/1, Product1/1

== system controller/Autonomous Controller/Throttle Command/Mux Everything/Build speed command ==
  CC : Inport  OutDataType=sfix(16)  OutScaling=2^0
  Constant : Constant  OutDataTypeMode=uint8  OutDataType=sfix(16)  OutScaling=2^0  OutDataTypeStr=uint8
  Constant1 : Constant  Value=0  OutDataTypeMode=uint8  OutDataType=sfix(16)  OutScaling=2^0  OutDataTypeStr=uint8
  Constant2 : Constant  Value=0  OutDataTypeMode=uint8  OutDataType=sfix(16)  OutScaling=2^0  OutDataTypeStr=uint8
  Constant3 : Constant  Value=5  OutDataTypeMode=uint8  OutDataType=sfix(16)  OutScaling=2^0  OutDataTypeStr=uint8
  Mux : Mux  Inputs=5
  uint16 to uchar : Subsystem  AncestorBlock=uSimLib/Conversions/uint16 to uchar
  msg : Outport  OutDataType=sfix(16)  OutScaling=2^0
  wires:
  CC/1 -> uint16 to uchar/1(ushort)
  Constant2/1 -> Mux/5
  Constant1/1 -> Mux/4
  Mux/1 -> msg/1
  Constant3/1 -> Mux/2
  Constant/1 -> Mux/1
  uint16 to uchar/1(uchar) -> Mux/3

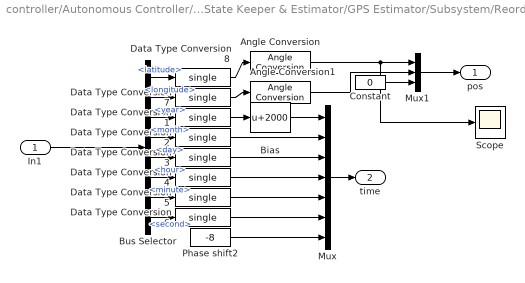
== system controller/Autonomous Controller/State Keeper & Estimator/GPS Estimator/Subsystem/Reorder ==
  In1 : Inport
  Angle Conversion : uSimLib/Conversions/Angle Conversion  SystemSampleTime=-1  iu=deg  ou=rad
  Angle Conversion1 : uSimLib/Conversions/Angle Conversion  SystemSampleTime=-1  iu=deg  ou=rad
  Bias : Bias  Bias=2000
  Bus Selector : BusSelector  OutputSignals=latitude,longitude,year,month,day,hour,minute,second
  Constant : Constant  Value=0  OutDataTypeMode=single  OutDataType=fixdt(1, 16)  OutScaling=2^0  OutDataTypeStr=single
  Data Type Conversion{1..8} (8 alike) : DataTypeConversion  OutDataTypeMode=single  OutDataType=fixdt(1, 16)  OutScaling=2^0  OutDataTypeStr=single
  Mux : Mux  Inputs=7
  Mux1 : Mux  Inputs=3
  Phase shift2 : Constant  Value=-8  OutDataTypeMode=single  OutDataType=sfix(16)  OutScaling=2^0  OutDataTypeStr=single
  Scope : Scope
  pos : Outport
  time : Outport  Port=2
  wires:
  Data Type Conversion8/1 -> Angle Conversion/1
  Data Type Conversion7/1 -> Angle Conversion1/1
  Mux1/1 -> pos/1
  Constant/1 -> Mux1/3
  Angle Conversion1/1 -> Mux1/2
  Angle Conversion/1 -> Mux1/1, Scope/1
  Mux/1 -> time/1
  In1/1 -> Bus Selector/1
  Phase shift2/1 -> Mux/7
  Data Type Conversion6/1 -> Mux/6
  Data Type Conversion5/1 -> Mux/5
  Data Type Conversion4/1 -> Mux/4
  Data Type Conversion3/1 -> Mux/3
  Bus Selector/8 -> Data Type Conversion6/1  "<second>"
  Bus Selector/7 -> Data Type Conversion5/1  "<minute>"
  Bus Selector/6 -> Data Type Conversion4/1  "<hour>"
  Bus Selector/5 -> Data Type Conversion3/1  "<day>"
  Bus Selector/4 -> Data Type Conversion2/1  "<month>"
  Bus Selector/3 -> Data Type Conversion1/1  "<year>"
  Data Type Conversion2/1 -> Mux/2
  Bias/1 -> Mux/1
  Data Type Conversion1/1 -> Bias/1
  Bus Selector/2 -> Data Type Conversion7/1  "<longitude>"
  Bus Selector/1 -> Data Type Conversion8/1  "<latitude>"

== system controller/Autonomous Controller/Throttle Command/Mux Everything/Build speed command/uint16 to uchar ==
  ushort : Inport
  Data Type Conversion : DataTypeConversion  OutDataTypeMode=uint16  OutDataType=fixdt(1, 16)  OutScaling=2^0  OutDataTypeStr=uint16  ConvertRealWorld=Stored Integer (SI)  RndMeth=Simplest
  Extract Bits1 : simulink/Logic and Bit Operations/Extract Bits  SystemSampleTime=-1  bitsToExtract=Upper half  numBits=8  bitIdxRange=[0 7]  outScalingMode=Treat bit field as an integer
  Extract Bits2 : simulink/Logic and Bit Operations/Extract Bits  SystemSampleTime=-1  bitsToExtract=Lower half  numBits=8  bitIdxRange=[0 7]  outScalingMode=Treat bit field as an integer
  Mux : Mux  Inputs=2
  uchar : Outport  OutDataType=fixdt(1, 16)  OutScaling=2^0
  wires:
  Data Type Conversion/1 -> Extract Bits2/1, Extract Bits1/1
  ushort/1 -> Data Type Conversion/1
  Extract Bits1/1 -> Mux/1
  Extract Bits2/1 -> Mux/2
  Mux/1 -> uchar/1

== matlab function Autonomous Controller/State Keeper & Estimator/GPS Estimator/Calculate local position via velocity integral between true GPS updates ==
  data: latLonAlt input single size=[3 1]; localPosition output single; newData input boolean size=1; reset input boolean size=1; resetIntegrator output boolean size=1
function [localPosition,resetIntegrator] = estimateGPS(latLonAlt, newData, reset)
%#eml
% INPUTS:
% latLonAlt - the latitude, longitude, and altitude of the vehicle from GPS
% newData - A boolean signal specifying whether latLonAlt holds new data
% reset - A global reset boolean trigger.

% OUTPUTS:
% localPosition is the local position of the vehicle in relation to a recorded
% starting location in North-East-Down coordinates.
% resetIntegrator will reset the velocity integrator that's calculating the
% local position in between GPS reads.

persistent startingPosition lastKnownPosition newDataCounter;

% Reset everything on first startup or when a global reset is triggered
if isempty(startingPosition) || reset
    startingPosition = zeros(3, 1, 'single');
end
if isempty(lastKnownPosition) || reset
    lastKnownPosition = zeros(3, 1, 'single');
end
if isempty(newDataCounter) || reset
    newDataCounter = zeros(1, 1, 'uint8');
end

% Reset the integrator if a global reset is called
if reset
    resetIntegrator = true;
else
    resetIntegrator = false;
end

% Wait for 5 valid GPS inputs before latching a starting point
if newDataCounter < 5
    % Check that we have valid data before latching it.
    if newData && latLonAlt(1) ~= 0 && latLonAlt(2) ~= 0
        newDataCounter = newDataCounter + 1;
        startingPosition = latLonAlt;
    end
    
    % We output all 0s while we're waiting
    localPosition = zeros(3, 1, 'single');
else
    % Latch a new position if one's been received. Also reset the integrator
    % for this timestep as we have a "truth" position now.
    if newData
        lastKnownPosition = latLonAlt;
        resetIntegrator = true;
    end
    
    % Calculate the difference between the starting position and the last
    % known position.
    localPosition = dg2lg(startingPosition, latLonAlt);
end

% Not certain how this works or where I got it from.
function out = dg2lg(u1, u2)

dlat = (u2(1) - u1(1))*pi/180;
dlon = (u2(2) - u1(2))*pi/180;
lat = u1(1)*pi/180;
h = u2(3);
a = 6378137;
e2 = 0.00669437999014;

v=a./sqrt(1-e2.*sin(lat).^2);
r=v.*(1-e2)./(1-e2.*sin(lat).^2);
dx=dlat.*(r+h);
dy=dlon.*cos(lat).*(v+h);

% Map into North-East-Down coordinates
out = [dy;-dx;0];

== matlab function Autonomous Controller/State Keeper & Estimator/GPS Estimator/Outputs/myMux1 ==
  data: u1 input double; y output double; u2 input double; u3 input double
function y = myMux(u1, u2, u3)
y = [u1(1); u2(1); u3(1)];

== matlab function Autonomous Controller/Rudder Command/L2 Plus ref WP1 ==
  data: reset input double; L2Vec output single; waypoints input int16; mode input uint8; Puav input single size=3; Vxyz input single size=3; switchDistance parameter double size=1; ISA_g parameter double; tanIntercept parameter double; MaxDwnPthStar parameter double; Turn2Track parameter double; InitialPoint parameter double; IPStar parameter double; TStar parameter double; as_c output single; i0 output double; i1 output double; WP0 output double; WP1 output double
function [L2Vec, as_c, i0, i1, WP0, WP1] = L2PlusWP1(reset, waypoints, mode, Puav, Vxyz, switchDistance, ...
    ISA_g, tanIntercept, MaxDwnPthStar,Turn2Track,...
    InitialPoint, IPStar, TStar)
%==============================
%     computes bank angle command for following a straight line
%     by creating an aim point that may be more than L2 away 
%     from the UAV. The aim point is (usually) farther along the path 
%     toward WP1 than the UAV, and the intercept
%     angle is less than or equal to a specified value. This limits the intercept
%     angle even when the UAV is within L2 of the path.
%     See L2PlusWP1.m for details
    
%         INPUTS   
%             T1      unit vector WP0-->WP1
%             N1      normal to T1
%             WP0     position of "from" waypoint. only needed to set an InitialPoint
%             WP1     position of WP1, active waypoint
%             Puav    position of UAV
%             Vxyz    Inertial velocity
%             switchDistance distance from WP1 to switch to WP2

%         PARAMETERS
%             ISA_g   gravity
%             tanIntercept  tangent of intercept angle
%             MaxDwnPthStar L2 multiplier to determmine downpath aimpoint
%             Turn2Track    true to turn toward T1 instead of L2
%             InitialPoint  true if no line tracking at first--fly direct to some initial point
%             IPStar        L2 multiplier to determing distance of IP from first WP0
%             Tstar         was called L2Base, time constant of response
%             
%         OUTPUTS
%             phi_c   commanded bank angle (positive is a starboard turn)
%             L2Vec   L2 vector toward aim point
%             as_c    commanded lateral acceleration
%             Groundspeed 
%             IP1     position of IP for plotting purposes. IP1(3) = -999 if no IP exists

    persistent IPActive;  %true if flying toward IP
    persistent IP; % location of initial point

    persistent index_0 index_1; % Store the indices for waypoints 0 & 1 respectively
    persistent direction; % Keep track of the direction for patrol mode
    
    % Make sure we have at least two waypoints
    assert(size(waypoints,1) >= 2);

    % Inititalize to the first waypoint
    if isempty(index_0)
        index_0 = int8(1);
    end
    if isempty(index_1)
        index_1 = int8(2);
    end
    if isempty(direction)
        direction = int8(1);
    end
    
    % Reset the waypoints
    if (reset)
        index_0 = int8(1);
        index_1 = int8(2);
    end
    
    % Select the two current waypoints we're dealing with
    WP0 = single(waypoints(index_0,:)');
    WP1 = single(waypoints(index_1,:)');
    i0 = index_0;
    i1 = index_1;
    
    switchToNextWaypoint = false;
    Pwp1 = single(zeros(3,1));
    Pe_y = single(0);
    Dist2WP1 = single(0);
    MinDownPath = single(0);
    Dist2WPSwitch = single(0);
    L2DownPath = single(0);
    L2ToT = single(zeros(3,1));
    L2Vec = single(zeros(3,1));
    IP1 = single([0; 0;-999]); %signal for no IP
    
    Pne = [Puav(1); Puav(2); 0]; %horizontal position
    Vne = [Vxyz(1); Vxyz(2); 0]; % horizontal velocity
    Groundspeed = norm(Vne);
    L2 = single(TStar*Groundspeed);
    WP0ne = single(zeros(3,1));
    
% Calculate N1 and T1
assert(norm(WP1 - WP0) ~= 0);
T1 = WP1-WP0;
T1 = T1/norm(T1);
N1 = [-T1(2); T1(1); 0];
    
%     initialize IP
    if (isempty(IPActive))
        if (InitialPoint)
%             IP is set relative to the first "from" waypoint
            IPActive = -1;
            IP = [WP0(1); WP0(2); 0] - L2*IPStar*T1;
            
            if (norm(IP-Pne) < .001)
                IPActive = 0;
                IP = single([0; 0; -999]);
            end
        else
            IPActive = 0;
            IP = single([0; 0;-999]); %signal for no IP
        end
    end
    IP1 = IP;
    
    
    if (IPActive)
%         no line tracking, direct to IP
        L2Vec = L2*(IP - Pne)/norm(IP - Pne);
%         check to see if at the IP to terminate this mode
        if norm(IP - Pne) < .1*L2
            IPActive = 0;
        end
    else
         if (Pne(1) < 2)
             IP1 = IP1;
         end
%         IP not active, track WP lines
        WPOne = [WP1(1); WP1(2); 0];
        Pwp1 = Pne - [WP1(1); WP1(2); 0]; % position of UAV relative to WP1
        Pe_y = single(Pwp1'*N1); % cross track error
        Dist2WP1 = -single(Pwp1'*T1); % distance to WP1

%         minimum down path distance for Aim Point intersection on T
%         is determined by the intercept angle but limited 
%         in case of very distant intecepts to MaxDwnPthStar*L2
        MinDownPath = single ( min( abs(Pe_y)/tanIntercept, MaxDwnPthStar*L2)); 
        Dist2WPSwitch = Dist2WP1 - switchDistance;
        if ( abs(Pe_y) > L2 )
    %             Make sure aimpoint is no closer to waypoint than calculated switch point.
            L2DownPath = MinDownPath;
        else
    %             within L2 of T and Dist2WPSwitch >= 0, but limit angle of L2 wrt T
            L2DownPath = (max(MinDownPath, (sqrt( L2^2 - Pe_y^2 ))));
        end
        
        if ( Dist2WPSwitch < 0 )
            switchToNextWaypoint = true;
        end
        
         % vector from Pwp1 to aim point on T1
         L2ToT = single(( Dist2WP1 - L2DownPath )*(-T1) - Pwp1);
         if (norm(L2ToT) < .001)
             L2Vec = L2*T1;
         else
            L2Vec = single(L2*( L2ToT/norm(L2ToT) )); % limit size to L2
         end
    %         L2Vec = L2ToT;
%         dummy statements
    end
    Zprod = single(Vxyz(1)*L2Vec(2) - Vxyz(2)*L2Vec(1)); %Z component of cross product
    sinEta = single(Zprod/(Groundspeed*L2));

    as_c = single(2*Groundspeed^2/(L2)*sinEta);
%         bank angle limits outside of this block
    phi_c = single(atan(as_c/ISA_g));

%         now override bank angle if heading in the wrong direction
    if ( Turn2Track && Dist2WPSwitch > 0 && ~IPActive ) 
%             turn to track not L2, gives min displacement from track
        if ( T1'*Vxyz < 0 )
            if ( Pe_y > 0 )
                phi_c = single(+pi/2);
                as_c = single(99);
            else
                phi_c = single(-pi/2);
                as_c = single(-99);
            end
        end
     else
%           turn toward L2, give min displacement toward WP0
        if ( L2Vec'*Vxyz < 0 )
            if ( sinEta < 0 )
                phi_c = single(-pi/2); 
                as_c = single(-99);
            else
                phi_c = single(+pi/2);
                as_c = single(99);
            end
        end
    end

% Now we process waypoint switching. This relies on the switchTrigger
% value set in the above L2+ controller code.
theEnd = false;
if index_1 + 1 <= size(waypoints,1) && waypoints(index_1+1,1) == -1 ...
                                    && waypoints(index_1+1,2) == -1 ...
                                    && waypoints(index_1+1,3) == -1
    theEnd = true;
end
if switchToNextWaypoint
    switch mode
        case 0 % Halt mode
            if size(waypoints,1) >= index_1 + 1 && ~theEnd
                index_0 = index_1;
                index_1 = index_1 + 1;
            end
        case 1 % Loop mode
            % We either continue moving forward through the waypoints...
            if size(waypoints,1) >= index_1 + 1 && ~theEnd
                index_0 = index_1;
                index_1 = index_1 + 1;
            % Or we wrap-around to the starting waypoint
            else
                index_0 = index_1;
                index_1 = int8(1);
            end
        case 2 % Patrol mode
            if direction == 1 % For the forwards direction
                % We either continue moving forwards through the waypoints...
                if size(waypoints,1) >= index_1 + 1 && ~theEnd
                    index_0 = index_1;
                    index_1 = index_1 + 1;
                % Or we start to go backwards
                else
                    index_0 = index_1;
                    index_1 = index_1 - 1;
                    direction = int8(0);
                end
            elseif direction == 0 % For the reverse direction
                % We either continue moving backwards through the waypoints...
                if index_1 - 1 >= 1
                    index_0 = index_1;
                    index_1 = index_1 - 1;
                % Or we start to go forwards
                else
                    index_0 = index_1;
                    index_1 = index_1 + 1;
                    direction = int8(1);
                end
            end
    end
end

== matlab function Autonomous Controller/Rudder Command/Embedded MATLAB Function ==
  data: u input double; y output double
function y = fcn(u)
%#eml

y = atan2(u(2), u(1)) * 180 / pi;

== matlab function Autonomous Controller/Throttle Command/Mux Everything/Select data packet ==
  data: y output double; dis input double; en input double
function y = fcn(dis, en)
% This block controls the switch selecting between enable, 
% disable, and speed commands. If disable and enable are
% both set high, disable overrides anything else.

y = uint8(3);
if dis == 1
    y = uint8(1);
elseif en == 1
    y = uint8(2);
end
